simulink model "Task08"  (R2022b)
settings: Solver=VariableStepAuto  StartTime=0.0  StopTime=10.0  RelTol=1e-3
settings Model: Creator=LOQ  LastModifiedBy=LOQ
settings OptimizationCC: ReuseModelBlockBuffer=on
settings RTWCC: GPUComputeCapability=5.0
settings ConfigComp: CovBoundaryAbsTol=1.0e-5

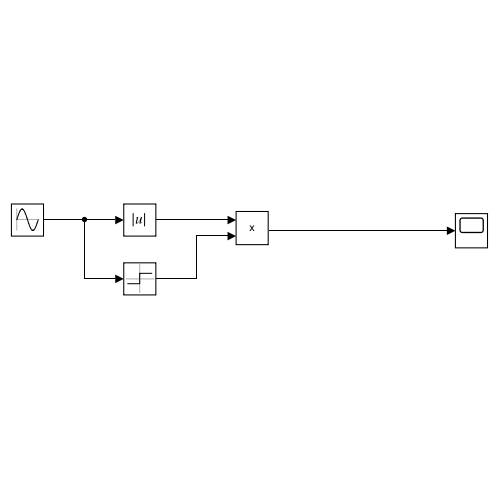
[thumbnail: Simulink's stored preview of the top-level diagram]
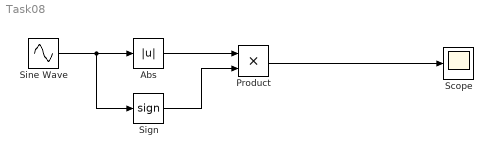
== system Task08 ==
  Abs : Abs  SaturateOnIntegerOverflow=off
  Product : Product
  Scope : Scope
  Sign : Signum
  Sine Wave : Sin  SampleTime=0
  wires:
  Sine Wave/1 -> Sign/1, Abs/1
  Abs/1 -> Product/1
  Sign/1 -> Product/2
  Product/1 -> Scope/1
